simulink model "Progetto_a1_simulink"  (R2022b)
settings: Solver=VariableStepAuto  StartTime=0.0  StopTime=100  RelTol=1e-3
values from neighbouring files (symbols this model uses):
  DD_ampiezza = 0.3    [Progetto_a1.m]
  DD_frequenza = 0.025    [Progetto_a1.m]
  denR = deR{1}    [Progetto_a1.m]
  NN_ampiezza = 0.2    [Progetto_a1.m]
  NN_frequenza = 1e3    (= 1000)    [Progetto_a1.m]
  numR = nuR{1}    [Progetto_a1.m]
  u_e = 2.17    [Progetto_a1.m]
  WW = 2    [Progetto_a1.m]
  x = [1,2,3,4]    [Progetto_a1.m]
  x01 = theta_e    (= 1.0471975512)    [Progetto_a1.m]
  x02 = 0    [Progetto_a1.m]
  ye = x01    (= 1.0471975512)    [Progetto_a1.m]
settings Model: Creator=anton  LastModifiedBy=anton

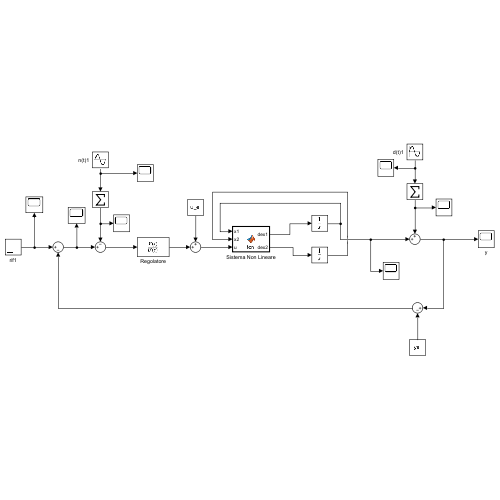
[thumbnail: Simulink's stored preview of the top-level diagram]
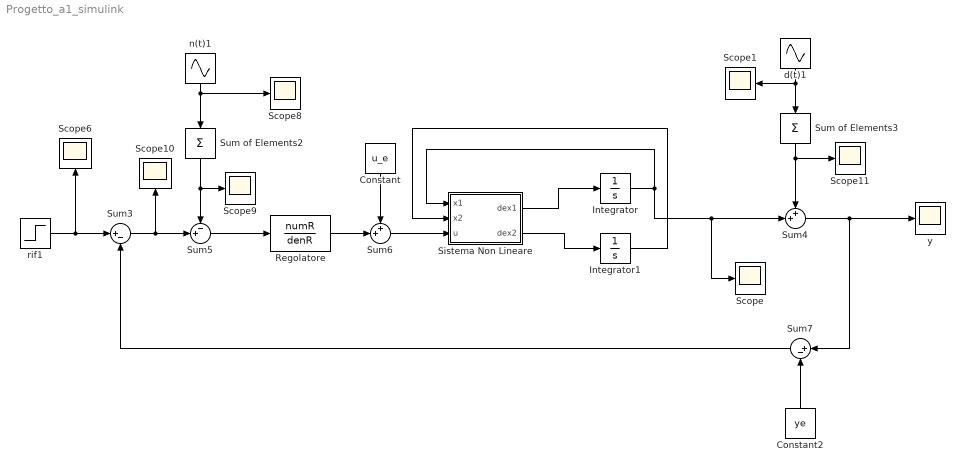
== system Progetto_a1_simulink ==
  Constant : Constant  Value=u_e
  Constant2 : Constant  Value=ye
  Integrator : Integrator  InitialCondition=x01
  Integrator1 : Integrator  InitialCondition=x02
  Regolatore : TransferFcn  Numerator=numR  Denominator=denR
  Scope{,1,6,8..11} (7 alike) : Scope
  Sistema Non Lineare : MATLAB Function  TreatAsAtomicUnit=on
  Sum of Elements2 : Sum  Inputs=+  CollapseDim=4
  Sum of Elements3 : Sum  Inputs=+  CollapseDim=4
  Sum3 : Sum  Inputs=|+-
  Sum4 : Sum  Inputs=++|
  Sum5 : Sum  Inputs=-+|
  Sum6 : Sum  Inputs=++|
  Sum7 : Sum  Inputs=|+-
  d(t)1 : Sin  Amplitude=DD_ampiezza  Frequency=DD_frequenza*x  SampleTime=0
  n(t)1 : Sin  Amplitude=NN_ampiezza  Frequency=NN_frequenza*x  SampleTime=0
  rif1 : Step  Time=0  After=WW  SampleTime=0
  y : Scope
  wires:
  Sistema Non Lineare/1(dex1) -> Integrator/1
  Sistema Non Lineare/2(dex2) -> Integrator1/1
  Integrator/1 -> Sistema Non Lineare/1(x1), Sum4/2, Scope/1
  Integrator1/1 -> Sistema Non Lineare/2(x2)
  Sum6/1 -> Sistema Non Lineare/3(u)
  Constant/1 -> Sum6/1
  Regolatore/1 -> Sum6/2
  Sum of Elements2/1 -> Sum5/1, Scope9/1
  Sum7/1 -> Sum3/2
  Sum5/1 -> Regolatore/1
  n(t)1/1 -> Sum of Elements2/1, Scope8/1
  Sum3/1 -> Scope10/1, Sum5/2
  rif1/1 -> Scope6/1, Sum3/1
  Constant2/1 -> Sum7/2
  Sum4/1 -> y/1, Sum7/1
  d(t)1/1 -> Sum of Elements3/1, Scope1/1
  Sum of Elements3/1 -> Sum4/1, Scope11/1

== matlab function Progetto_a1_simulink/Sistema Non Lineare ==
  data: x1 input; x2 input; u input; dex1 output; dex2 output
function [dex1,dex2] = fcn(x1,x2,u)
% Parametri
beta = 0.5;
J = 10;
a = 0.01;
F_v = -5;

dex1 = x2;
dex2 = (-beta/J)*x2+(a/(2*J))*sin(x1)*F_v+(a/J)*u;
